simulink model "validation_of_rotation_component"  (R2019b)
settings: Solver=VariableStepAuto  StartTime=0.0  StopTime=10.0  RelTol=1e-3
undefined symbols (not defined in the file): r
settings Model: Creator=chiragg  LastModifiedBy=chiragg

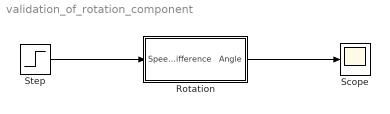
== system validation_of_rotation_component ==
  Rotation : Subsystem
  Scope : Scope
  Step : Step  SampleTime=0
  wires:
  Step/1 -> Rotation/1(Speed difference)
  Rotation/1(Angle) -> Scope/1

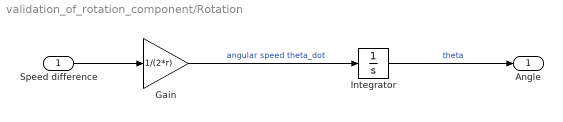
== system validation_of_rotation_component/Rotation ==
  Speed difference : Inport
  Gain : Gain  Gain=1/(2*r)
  Integrator : Integrator
  Angle : Outport
  wires:
  Speed difference/1 -> Gain/1
  Gain/1 -> Integrator/1  "angular speed theta_dot"
  Integrator/1 -> Angle/1  "theta"
